simulink model "AAI"  (R2020a)
settings: Solver=VariableStepAuto  StartTime=0.0  StopTime=10.0  RelTol=1e-3
undefined symbols (not defined in the file): D0, D10, D11, D13, D2, D3, D4, D5, D6, D8, PTA0, PTA1, PTA2, PTB23, PTB9, PTC16, PTC2, PTD0, PTD1, PTD2
libraries: frdmk64flib x10
settings Model: Creator=amnay  LastModifiedBy=amnay

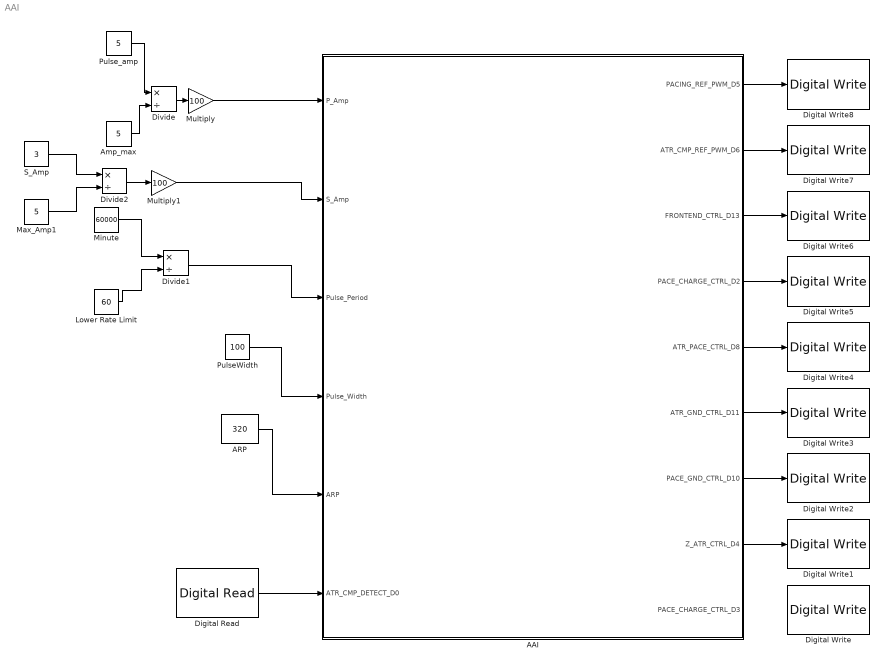
== system AAI ==
  AAI : Stateflow chart  TreatAsAtomicUnit=on
  ARP : Constant  Value=320
  Amp_max : Constant  Value=5
  Digital Read : frdmk64flib/Digital Read  Whichpin=PTC16 (D0)  SampleTime=-1
  Digital Write : frdmk64flib/Digital Write  Whichpin=PTA1 (D3)
  Digital Write1 : frdmk64flib/Digital Write  Whichpin=PTB23 (D4)
  Digital Write2 : frdmk64flib/Digital Write  Whichpin=PTD0 (D10)
  Digital Write3 : frdmk64flib/Digital Write  Whichpin=PTD2 (D11)
  Digital Write4 : frdmk64flib/Digital Write  Whichpin=PTA0 (D8)
  Digital Write5 : frdmk64flib/Digital Write  Whichpin=PTB9 (D2)
  Digital Write6 : frdmk64flib/Digital Write  Whichpin=PTD1 (D13)
  Digital Write7 : frdmk64flib/Digital Write  Whichpin=PTC2 (D6)
  Digital Write8 : frdmk64flib/Digital Write  Whichpin=PTA2 (D5)
  Divide : Product  Inputs=*/
  Divide1 : Product  Inputs=*/
  Divide2 : Product  Inputs=*/
  Lower Rate Limit : Constant  Value=60
  Max_Amp1 : Constant  Value=5
  Minute : Constant  Value=60000
  Multiply : Gain  Gain=100
  Multiply1 : Gain  Gain=100
  PulseWidth : Constant  Value=100
  Pulse_amp : Constant  Value=5
  S_Amp : Constant  Value=3
  wires:
  Multiply/1 -> AAI/1(P_Amp)
  Divide/1 -> Multiply/1
  Pulse_amp/1 -> Divide/1
  Amp_max/1 -> Divide/2
  Minute/1 -> Divide1/1
  Lower Rate Limit/1 -> Divide1/2
  Max_Amp1/1 -> Divide2/2
  S_Amp/1 -> Divide2/1
  Divide2/1 -> Multiply1/1
  Divide1/1 -> AAI/3(Pulse_Period)
  Multiply1/1 -> AAI/2(S_Amp)
  PulseWidth/1 -> AAI/4(Pulse_Width)
  ARP/1 -> AAI/5(ARP)
  Digital Read/1 -> AAI/6(ATR_CMP_DETECT_D0)
  AAI/8(Z_ATR_CTRL_D4) -> Digital Write1/1
  AAI/7(PACE_GND_CTRL_D10) -> Digital Write2/1
  AAI/6(ATR_GND_CTRL_D11) -> Digital Write3/1
  AAI/5(ATR_PACE_CTRL_D8) -> Digital Write4/1
  AAI/4(PACE_CHARGE_CTRL_D2) -> Digital Write5/1
  AAI/3(FRONTEND_CTRL_D13) -> Digital Write6/1
  AAI/2(ATR_CMP_REF_PWM_D6) -> Digital Write7/1
  AAI/1(PACING_REF_PWM_D5) -> Digital Write8/1

== stateflow chart AAI/AAI ==
  state AAI_Charging_Sensing
    entry:
    PACING_REF_PWM_D5= P_Amp;
    ATR_CMP_REF_PWM_D6= S_Amp;
    FRONTEND_CTRL_D13= 1;
    PACE_CHARGE_CTRL_D2 = 1;
    ATR_PACE_CTRL_D8 = 0;
    ATR_GND_CTRL_D11= 1;
    PACE_GND_CTRL_D10= 0;
    Z_ATR_CTRL_D4= 0;
  state AAI_Pacing
    entry:
    PACING_REF_PWM_D5= P_Amp;
    PACE_CHARGE_CTRL_D2 = 0;
    ATR_PACE_CTRL_D8 = 1;
    ATR_GND_CTRL_D11= 0;
    Z_ATR_CTRL_D4 = 0;
  state AAI_Discharging
    entry:
    PACE_GND_CTRL_D10 = 1;
    ATR_PACE_CTRL_D8= 0;
    ATR_GND_CTRL_D11 = 1;
    Z_ATR_CTRL_D4= 0;
  (default) -> AAI_Charging_Sensing
  AAI_Charging_Sensing -> AAI_Pacing
  AAI_Pacing -> AAI_Discharging
  AAI_Discharging -> AAI_Charging_Sensing
  data: P_Amp input; S_Amp input; Pulse_Period input; Pulse_Width input; ARP input; ATR_CMP_DETECT_D0 input; PACING_REF_PWM_D5 output; ATR_CMP_REF_PWM_D6 output; FRONTEND_CTRL_D13 output; PACE_CHARGE_CTRL_D2 output; ATR_PACE_CTRL_D8 output; ATR_GND_CTRL_D11 output; PACE_GND_CTRL_D10 output; Z_ATR_CTRL_D4 output; PACE_CHARGE_CTRL_D3 output
